simulink library "walkingRobotUtils"  (R2019b)
settings: Solver=VariableStepAuto  StartTime=0.0  StopTime=10.0  RelTol=1e-3
undefined symbols (not defined in the file): ankle_servo_kd, ankle_servo_ki, ankle_servo_kp, deriv_filter_coeff, foot_x, foot_y, foot_z, height_plane, hip_servo_kd, hip_servo_ki, hip_servo_kp, init_angs_L, init_angs_R, init_height, joint_damping, knee_servo_kd, knee_servo_ki, knee_servo_kp, leg_width, lower_leg_length, max_torque, motion_time_constant, motor_constant, motor_inertia, motor_voltage, plane_x, plane_y, plane_z, torso_height, torso_length, torso_offset_height, torso_offset_length, torso_offset_x, torso_offset_z, torso_width, torso_x, torso_y, torso_z, upper_leg_length, X, Y, Z
libraries: sm_lib x116, nesl_utility x49, $bdroot x33, simulink x33, simulink_extras x32, fl_lib x7, ee_lib x3, Multibody_Multiphysics_Lib x1
(part 1 of 6)
settings Model: Creator=scastro  LastModifiedBy=scastro
settings DataIOCC: ReturnWorkspaceOutputs=off
settings DebuggingCC: ArithmeticOperatorsInVariantConditions=warning
settings SFSimCC: SimUseLocalCustomCode=off  CustomCodeUndefinedFunction=UseInterfaceOnly
settings RTWCC: RTWUseLocalCustomCode=off
settings CodeAppCC: StateflowObjectComments=on

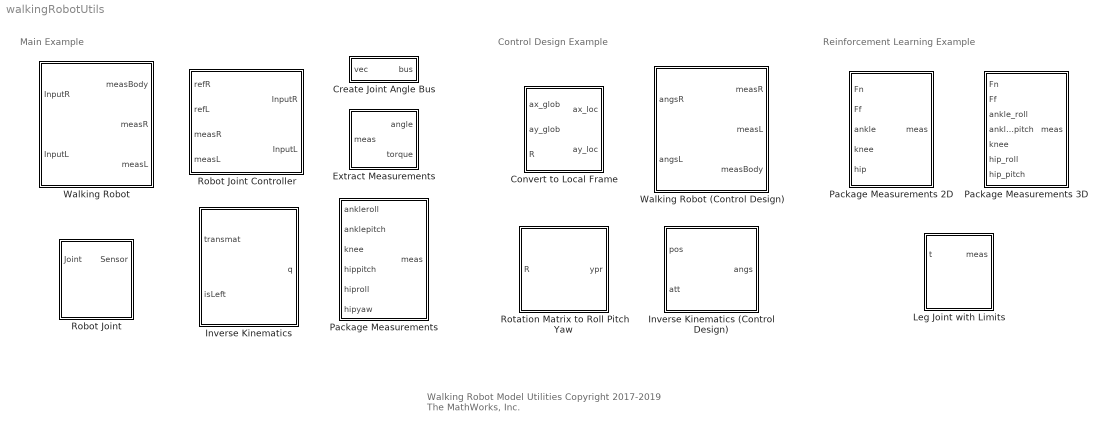
== system walkingRobotUtils ==
  note: Reinforcement Learning Example
  note: Control Design Example
  note: Main Example
  note: Walking Robot Model Utilities
      |
      | Copyright 2017-2019 The MathWorks, Inc.
  Convert to Local Frame : Subsystem
  Create Joint Angle Bus : Subsystem
  Extract Measurements : Subsystem
  Inverse Kinematics : MATLAB Function  TreatAsAtomicUnit=on
  Inverse Kinematics (Control Design) : MATLAB Function  TreatAsAtomicUnit=on
  Leg Joint with Limits : Subsystem  VariantControl=actuatorType == 2  mask(Leg Joint with Limits){k=1, d=0, initAngle=0, eqAngle=0, upperLimit=0, lowerLimit=-pi/8, jointLimitStiffness=100, jointLimitDamping=10}
      mask prompts: k "Joint Stiffness [N*m/rad]"; d "Joint Damping [N*m/(rad/s)]"; initAngle "Initial Angle [rad]"; eqAngle "Equilibrium Angle [rad]"; upperLimit "Upper Angle Limit [rad]"; lowerLimit "Lower Angle Limit [rad]"; jointLimitStiffness "Joint Limit Stiffness [N*m/rad]"; jointLimitDamping "Joint Limit Damping [N*m/(rad/s)]"
      mask help: Torque-actuated revolute joint with limits and instrumented measurements.
      mask DialogControl DynamicsTab Prompt: Dynamics
      mask DialogControl LimitsTab Prompt: Limits
  Package Measurements 3D : Subsystem
  Package Measurements 2D : Subsystem
  Package Measurements : Subsystem
  Robot Joint : Subsystem  Variant=on  mask{jointDamping=joint_damping, initAngle=0, upperLimit=pi/2, lowerLimit=-pi/2, limitK=1000, limitD=100}
      mask prompts: jointDamping "Joint Damping [N*m/(rad/s)"; initAngle "Initial Angle [rad]"; upperLimit "Upper Angle Limit [rad]"; lowerLimit "Lower Angle Limit [rad]"; limitK "Joint Limit Stiffness [N*m/rad]"; limitD "Joint Limit Damping [N*m/(rad/s)"
      mask help: Joint and actuator for walking robot example.
  Robot Joint Controller : Subsystem  Variant=on
  Rotation Matrix to Roll Pitch Yaw : MATLAB Function  TreatAsAtomicUnit=on
  Walking Robot : Subsystem
  Walking Robot (Control Design) : Subsystem

== system walkingRobotUtils/Convert to Local Frame ==
  ax_glob : Inport
  ay_glob : Inport  Port=2
  R : Inport  Port=3
  Constant : Constant  Value=0
  Demux1 : Demux  Outputs=2
  Matrix Multiply : Product  Multiplication=Matrix(*)
  Mux : Mux  Inputs=3
  Selector : Selector  InputPortWidth=3  IndexOptions=Index vector (dialog)  Indices=[1 2]  OutputSizes=1
  Transpose : Math  Operator=transpose  SaturateOnIntegerOverflow=on
  ax_loc : Outport  VectorParamsAs1DForOutWhenUnconnected=off
  ay_loc : Outport  Port=2  VectorParamsAs1DForOutWhenUnconnected=off
  wires:
  Mux/1 -> Matrix Multiply/2
  Demux1/2 -> ay_loc/1
  ay_glob/1 -> Mux/2
  Selector/1 -> Demux1/1
  Matrix Multiply/1 -> Selector/1
  Constant/1 -> Mux/3
  ax_glob/1 -> Mux/1
  Demux1/1 -> ax_loc/1
  R/1 -> Transpose/1
  Transpose/1 -> Matrix Multiply/1

== system walkingRobotUtils/Create Joint Angle Bus ==
  vec : Inport
  Bus Creator : BusCreator  Inputs=6
  Demux : Demux  Outputs=6
  Gain : Gain  Gain=-1
  Gain1 : Gain  Gain=-1
  Gain2 : Gain  Gain=-1
  bus : Outport  VectorParamsAs1DForOutWhenUnconnected=off
  wires:
  Gain2/1 -> Bus Creator/5  "ankle pitch"
  Gain1/1 -> Bus Creator/4  "knee"
  Demux/5 -> Gain2/1
  vec/1 -> Demux/1
  Demux/4 -> Gain1/1
  Bus Creator/1 -> bus/1
  Gain/1 -> Bus Creator/3  "hip pitch"
  Demux/1 -> Bus Creator/1  "hip yaw"
  Demux/6 -> Bus Creator/6  "ankle roll"
  Demux/2 -> Bus Creator/2  "hip roll"
  Demux/3 -> Gain/1

== system walkingRobotUtils/Extract Measurements ==
  meas : Inport
  Bus Selector : BusSelector  OutputSignals=angle,torque
  angle : Outport  VectorParamsAs1DForOutWhenUnconnected=off
  torque : Outport  Port=2  VectorParamsAs1DForOutWhenUnconnected=off
  wires:
  Bus Selector/1 -> angle/1  "<angle>"
  meas/1 -> Bus Selector/1
  Bus Selector/2 -> torque/1  "<torque>"

== system walkingRobotUtils/Leg Joint with Limits ==
  t : Inport
  Bus Creator : BusCreator  Inputs=3
  PS-Simulink Converter1 : nesl_utility/PS-Simulink Converter  PhysicalDomain=network_engine_domain  SubClassName=ps_output  LeftPortType=input  RightPortType=output  PseudoPeriodic=off  Frequencies=[]  Unit=rad  AffineConversion=off
  PS-Simulink Converter2 : nesl_utility/PS-Simulink Converter  PhysicalDomain=network_engine_domain  SubClassName=ps_output  LeftPortType=input  RightPortType=output  PseudoPeriodic=off  Frequencies=[]  Unit=rad/s  AffineConversion=off
  Revolute Joint : sm_lib/Joints/Revolute Joint  JointMode=Normal  SenseConstraintForce=off  SenseConstraintForceX=off  SenseConstraintForceY=off  SenseConstraintForceZ=off  SenseConstraintTorque=off  SenseConstraintTorqueX=off  SenseConstraintTorqueY=off  SenseConstraintTorqueZ=off  SenseTotalForce=off  SenseTotalForceX=off  SenseTotalForceY=off  SenseTotalForceZ=off  SenseTotalTorque=off  SenseTotalTorqueX=off  SenseTotalTorqueY=off  SenseTotalTorqueZ=off  CompositeWrenchDir=FollowerOnBase  CompositeWrenchFrame=BaseFrame  EquilibriumPosition=eqAngle  EquilibriumPositionUnits=rad  SpringStiffness=k  SpringStiffnessUnits=N*m/rad  DampingCoefficient=d  DampingCoefficientUnits=N*m/(rad/s)  TorqueActuationMode=InputTorque  MotionActuationMode=ComputedMotion  SensePosition=on  SenseVelocity=on  SenseAcceleration=off  SenseTorqueForce=off  SenseLowerLimitTorqueForce=off  SenseUpperLimitTorqueForce=off  LowerLimitSpecify=on  LowerLimitBound=lowerLimit  LowerLimitBoundUnits=rad  LowerLimitStiffness=jointLimitStiffness  LowerLimitStiffnessUnits=N*m/rad  LowerLimitDamping=jointLimitDamping  LowerLimitDampingUnits=N*m/(rad/s)  LowerLimitTransitionRegionWidth=1  LowerLimitTransitionRegionWidthUnits=deg  UpperLimitSpecify=on  UpperLimitBound=upperLimit  UpperLimitBoundUnits=rad  UpperLimitStiffness=jointLimitStiffness  UpperLimitStiffnessUnits=N*m/rad  UpperLimitDamping=jointLimitDamping  UpperLimitDampingUnits=N*m/(rad/s)  UpperLimitTransitionRegionWidth=1  UpperLimitTransitionRegionWidthUnits=deg  PositionTargetSpecify=on  PositionTargetPriority=High  PositionTargetValue=initAngle  PositionTargetValueUnits=rad  VelocityTargetSpecify=off  VelocityTargetPriority=High  VelocityTargetValue=0  VelocityTargetValueUnits=deg/s
  Simulink-PS Converter : nesl_utility/Simulink-PS Converter  PhysicalDomain=network_engine_domain  SubClassName=ps_input  LeftPortType=input  RightPortType=output  PseudoPeriodic=off  Frequencies=[]  NoiseDistribution=none  NoiseParameters=[]  Unit=N*m  AffineConversion=off  FilteringAndDerivatives=provide  SimscapeFilterOrder=2  InputFilterTimeConstant=motion_time_constant  UdotUserProvided=0
  B : PMIOPort  Side=Left
  F : PMIOPort  Port=2  Side=Right
  meas : Outport  VectorParamsAs1DForOutWhenUnconnected=off
  wires:
  PS-Simulink Converter2/1 -> Bus Creator/3  "speed"
  t/1 -> Simulink-PS Converter/1, Bus Creator/1  "torque"
  Bus Creator/1 -> meas/1
  PS-Simulink Converter1/1 -> Bus Creator/2  "angle"
  connections:
  PS-Simulink Converter2/LConn1 -- Revolute Joint/RConn3
  Simulink-PS Converter/RConn1 -- Revolute Joint/LConn2
  Revolute Joint/RConn1 -- F/RConn1
  Revolute Joint/LConn1 -- B/RConn1
  PS-Simulink Converter1/LConn1 -- Revolute Joint/RConn2

== system walkingRobotUtils/Package Measurements 3D ==
  Fn : Inport
  Ff : Inport  Port=2
  ankle_roll : Inport  Port=3
  ankle_pitch : Inport  Port=4
  knee : Inport  Port=5
  hip_roll : Inport  Port=6
  hip_pitch : Inport  Port=7
  Bus Creator3 : BusCreator  Inputs=17
  Extract Measurements : Subsystem
  Extract Measurements1 : Subsystem
  Extract Measurements2 : Subsystem
  Extract Measurements3 : Subsystem
  Extract Measurements4 : Subsystem
  meas : Outport  VectorParamsAs1DForOutWhenUnconnected=off
  wires:
  Extract Measurements4/2(speed) -> Bus Creator3/16  "hip_pitch_speed"
  Extract Measurements3/2(speed) -> Bus Creator3/13  "hip_roll_speed"
  Extract Measurements2/2(speed) -> Bus Creator3/10  "knee_speed"
  Extract Measurements2/1(angle) -> Bus Creator3/9  "knee_angle"
  Extract Measurements1/2(speed) -> Bus Creator3/7  "ankle_pitch_speed"
  Extract Measurements/2(speed) -> Bus Creator3/4  "ankle_roll_speed"
  Fn/1 -> Bus Creator3/1  "normal_force"
  Ff/1 -> Bus Creator3/2  "friction_force"
  Extract Measurements4/3(torque) -> Bus Creator3/17  "hip_pitch_torque"
  Extract Measurements4/1(angle) -> Bus Creator3/15  "hip_pitch_angle"
  Extract Measurements2/3(torque) -> Bus Creator3/11  "knee_torque"
  hip_pitch/1 -> Extract Measurements4/1(meas)
  knee/1 -> Extract Measurements2/1(meas)
  Extract Measurements1/3(torque) -> Bus Creator3/8  "ankle_pitch_torque"
  Extract Measurements1/1(angle) -> Bus Creator3/6  "ankle_pitch_angle"
  ankle_pitch/1 -> Extract Measurements1/1(meas)
  Bus Creator3/1 -> meas/1
  ankle_roll/1 -> Extract Measurements/1(meas)
  Extract Measurements/1(angle) -> Bus Creator3/3  "ankle_roll_angle"
  Extract Measurements/3(torque) -> Bus Creator3/5  "ankle_roll_torque"
  hip_roll/1 -> Extract Measurements3/1(meas)
  Extract Measurements3/3(torque) -> Bus Creator3/14  "hip_roll_torque"
  Extract Measurements3/1(angle) -> Bus Creator3/12  "hip_roll_angle"

== system walkingRobotUtils/Package Measurements 2D ==
  Fn : Inport
  Ff : Inport  Port=2
  ankle : Inport  Port=3
  knee : Inport  Port=4
  hip : Inport  Port=5
  Bus Creator3 : BusCreator  Inputs=11
  Extract Measurements : Subsystem
  Extract Measurements1 : Subsystem
  Extract Measurements2 : Subsystem
  meas : Outport  VectorParamsAs1DForOutWhenUnconnected=off
  wires:
  Extract Measurements2/2(speed) -> Bus Creator3/10  "hip_speed"
  Extract Measurements1/2(speed) -> Bus Creator3/7  "knee_speed"
  Extract Measurements/2(speed) -> Bus Creator3/4  "ankle_speed"
  Bus Creator3/1 -> meas/1
  ankle/1 -> Extract Measurements/1(meas)
  Extract Measurements/1(angle) -> Bus Creator3/3  "ankle_angle"
  Extract Measurements/3(torque) -> Bus Creator3/5  "ankle_torque"
  knee/1 -> Extract Measurements1/1(meas)
  hip/1 -> Extract Measurements2/1(meas)
  Extract Measurements1/1(angle) -> Bus Creator3/6  "knee_angle"
  Extract Measurements1/3(torque) -> Bus Creator3/8  "knee_torque"
  Extract Measurements2/1(angle) -> Bus Creator3/9  "hip_angle"
  Extract Measurements2/3(torque) -> Bus Creator3/11  "hip_torque"
  Ff/1 -> Bus Creator3/2  "friction_force"
  Fn/1 -> Bus Creator3/1  "normal_force"

== system walkingRobotUtils/Package Measurements ==
  ankleroll : Inport
  anklepitch : Inport  Port=2
  knee : Inport  Port=3
  hippitch : Inport  Port=4
  hiproll : Inport  Port=5
  hipyaw : Inport  Port=6
  Bus Creator3 : BusCreator  Inputs=12
  Extract Measurements : Subsystem
  Extract Measurements{1..5} (5 alike) : $bdroot/Package Measurements/Extract Measurements  SystemSampleTime=-1  Latency=0  AutoFrameSizeCalculation=off
  meas : Outport  VectorParamsAs1DForOutWhenUnconnected=off
  wires:
  hiproll/1 -> Extract Measurements4/1
  Extract Measurements1/2 -> Bus Creator3/4  "anklepitch_torque"
  Bus Creator3/1 -> meas/1
  anklepitch/1 -> Extract Measurements1/1
  hippitch/1 -> Extract Measurements3/1
  hipyaw/1 -> Extract Measurements5/1
  Extract Measurements5/1 -> Bus Creator3/11  "hipyaw_angle"
  Extract Measurements/2(torque) -> Bus Creator3/2  "ankleroll_torque"
  Extract Measurements4/1 -> Bus Creator3/9  "hiproll_angle"
  knee/1 -> Extract Measurements2/1
  Extract Measurements2/1 -> Bus Creator3/5  "knee_angle"
  Extract Measurements/1(angle) -> Bus Creator3/1  "ankleroll_angle"
  ankleroll/1 -> Extract Measurements/1(meas)
  Extract Measurements3/2 -> Bus Creator3/8  "hippitch_torque"
  Extract Measurements1/1 -> Bus Creator3/3  "anklepitch_angle"
  Extract Measurements3/1 -> Bus Creator3/7  "hippitch_angle"
  Extract Measurements5/2 -> Bus Creator3/12  "hipyaw_torque"
  Extract Measurements2/2 -> Bus Creator3/6  "knee_torque"
  Extract Measurements4/2 -> Bus Creator3/10  "hiproll_torque"

== system walkingRobotUtils/Robot Joint ==
  note: 1) Add Subsystem or Model blocks as valid variant choices.
      | 2) You cannot connect blocks at this level. At simulation, connectivity is automatically
      | determined, based on the active variant and port name matching.
  Joint : Inport
  Motion : Subsystem  VariantControl=actuatorType == 1
  Motor : Subsystem  VariantControl=actuatorType == 3
  Torque : Subsystem  VariantControl=actuatorType == 2
  F : PMIOPort  Side=Right
  B : PMIOPort  Port=2  Side=Left
  Sensor : Outport  VectorParamsAs1DForOutWhenUnconnected=off

== system walkingRobotUtils/Robot Joint Controller ==
  note: 1) Add Subsystem or Model blocks as valid variant choices.
      | 2) You cannot connect blocks at this level. At simulation, connectivity is automatically
      | determined, based on the active variant and port name matching.
  refR : Inport
  refL : Inport  Port=2
  measR : Inport  Port=3
  measL : Inport  Port=4
  Motion : Subsystem  VariantControl=actuatorType == 1
  Motor : Subsystem  VariantControl=actuatorType == 3
  Torque : Subsystem  VariantControl=actuatorType == 2
  InputR : Outport  VectorParamsAs1DForOutWhenUnconnected=off
  InputL : Outport  Port=2  VectorParamsAs1DForOutWhenUnconnected=off

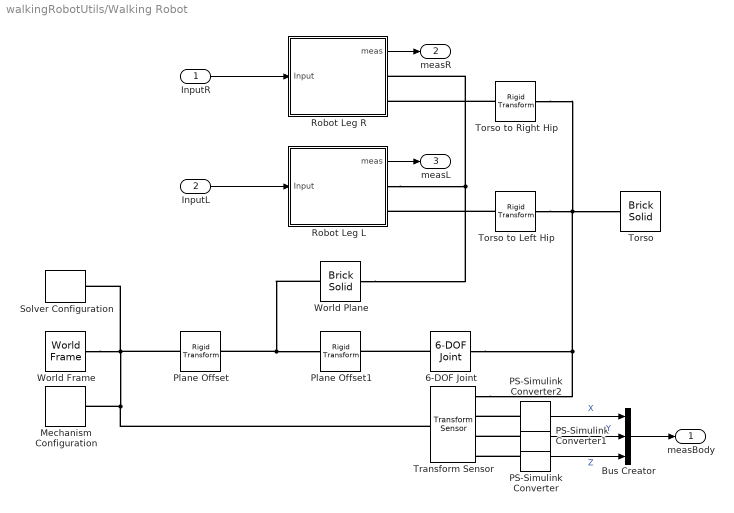
== system walkingRobotUtils/Walking Robot ==
  InputR : Inport
  InputL : Inport  Port=2
  6-DOF Joint : sm_lib/Joints/6-DOF Joint  JointMode=Normal  SenseConstraintForce=off  SenseConstraintForceX=off  SenseConstraintForceY=off  SenseConstraintForceZ=off  SenseConstraintTorque=off  SenseConstraintTorqueX=off  SenseConstraintTorqueY=off  SenseConstraintTorqueZ=off  SenseTotalForce=off  SenseTotalForceX=off  SenseTotalForceY=off  SenseTotalForceZ=off  SenseTotalTorque=off  SenseTotalTorqueX=off  SenseTotalTorqueY=off  SenseTotalTorqueZ=off  CompositeWrenchDir=FollowerOnBase  CompositeWrenchFrame=BaseFrame  PxEquilibriumPosition=0  PxEquilibriumPositionUnits=m  PxSpringStiffness=0  PxSpringStiffnessUnits=N/m  PxDampingCoefficient=world_damping  PxDampingCoefficientUnits=N/(m/s)  PxTorqueActuationMode=NoTorque  PxMotionActuationMode=ComputedMotion  PxSensePosition=off  PxSenseVelocity=off  PxSenseAcceleration=off  PxSenseTorqueForce=off  PxSenseLowerLimitTorqueForce=off  PxSenseUpperLimitTorqueForce=off  PxLowerLimitSpecify=off  PxLowerLimitBound=-1  PxLowerLimitBoundUnits=m  PxLowerLimitStiffness=1e6  PxLowerLimitStiffnessUnits=N/m  PxLowerLimitDamping=1e3  PxLowerLimitDampingUnits=N/(m/s)  PxLowerLimitTransitionRegionWidth=1e-4  PxLowerLimitTransitionRegionWidthUnits=m  PxUpperLimitSpecify=off  PxUpperLimitBound=1  PxUpperLimitBoundUnits=m  PxUpperLimitStiffness=1e6  PxUpperLimitStiffnessUnits=N/m  PxUpperLimitDamping=1e3  PxUpperLimitDampingUnits=N/(m/s)  PxUpperLimitTransitionRegionWidth=1e-4  PxUpperLimitTransitionRegionWidthUnits=m  PxPositionTargetSpecify=off  PxPositionTargetPriority=High  PxPositionTargetValue=0  PxPositionTargetValueUnits=m  PxVelocityTargetSpecify=off  PxVelocityTargetPriority=High  PxVelocityTargetValue=0  PxVelocityTargetValueUnits=m/s  PyEquilibriumPosition=0  PyEquilibriumPositionUnits=m  PySpringStiffness=0  PySpringStiffnessUnits=N/m  PyDampingCoefficient=world_damping  PyDampingCoefficientUnits=N/(m/s)  PyTorqueActuationMode=NoTorque  PyMotionActuationMode=ComputedMotion  PySensePosition=off  PySenseVelocity=off  PySenseAcceleration=off  PySenseTorqueForce=off  PySenseLowerLimitTorqueForce=off  PySenseUpperLimitTorqueForce=off  PyLowerLimitSpecify=off  PyLowerLimitBound=-1  PyLowerLimitBoundUnits=m  PyLowerLimitStiffness=1e6  PyLowerLimitStiffnessUnits=N/m  PyLowerLimitDamping=1e3  PyLowerLimitDampingUnits=N/(m/s)  PyLowerLimitTransitionRegionWidth=1e-4  PyLowerLimitTransitionRegionWidthUnits=m  PyUpperLimitSpecify=off  PyUpperLimitBound=1  PyUpperLimitBoundUnits=m  PyUpperLimitStiffness=1e6  PyUpperLimitStiffnessUnits=N/m  PyUpperLimitDamping=1e3  PyUpperLimitDampingUnits=N/(m/s)  PyUpperLimitTransitionRegionWidth=1e-4  PyUpperLimitTransitionRegionWidthUnits=m  PyPositionTargetSpecify=off  PyPositionTargetPriority=High  PyPositionTargetValue=0  PyPositionTargetValueUnits=m  PyVelocityTargetSpecify=off  PyVelocityTargetPriority=High  PyVelocityTargetValue=0  PyVelocityTargetValueUnits=m/s  PzEquilibriumPosition=0  PzEquilibriumPositionUnits=m  PzSpringStiffness=0  PzSpringStiffnessUnits=N/m  PzDampingCoefficient=world_damping  PzDampingCoefficientUnits=N/(m/s)  PzTorqueActuationMode=NoTorque  PzMotionActuationMode=ComputedMotion  PzSensePosition=off  PzSenseVelocity=off  PzSenseAcceleration=off  PzSenseTorqueForce=off  PzSenseLowerLimitTorqueForce=off  PzSenseUpperLimitTorqueForce=off  PzLowerLimitSpecify=off  PzLowerLimitBound=-1  PzLowerLimitBoundUnits=m  PzLowerLimitStiffness=1e6  PzLowerLimitStiffnessUnits=N/m  PzLowerLimitDamping=1e3  PzLowerLimitDampingUnits=N/(m/s)  PzLowerLimitTransitionRegionWidth=1e-4  PzLowerLimitTransitionRegionWidthUnits=m  PzUpperLimitSpecify=off  PzUpperLimitBound=1  PzUpperLimitBoundUnits=m  PzUpperLimitStiffness=1e6  PzUpperLimitStiffnessUnits=N/m  PzUpperLimitDamping=1e3  PzUpperLimitDampingUnits=N/(m/s)  PzUpperLimitTransitionRegionWidth=1e-4  PzUpperLimitTransitionRegionWidthUnits=m  PzPositionTargetSpecify=on  PzPositionTargetPriority=High  PzPositionTargetValue=init_height  PzPositionTargetValueUnits=m  PzVelocityTargetSpecify=off  PzVelocityTargetPriority=High  PzVelocityTargetValue=0  PzVelocityTargetValueUnits=m/s  SphDefPosRotationMethod=None  SphDefPosRotationAngleUnits=deg  SphDefPosRotationStandardAxis=+Z  SphDefPosRotationAngle=0.0  SphDefPosRotationArbitraryAxis=[0 0 1]  SphDefPosFollAlignAxisA=+X  SphDefPosBaseAlignAxisA=+Y  SphDefPosFollAlignAxisB=+Y  SphDefPosBaseAlignAxisB=+Z  SphDefPosRotationSequenceAxes=FollowerAxes  SphDefPosRotationSequence=XYX  SphDefPosRotationSequenceAngles=[0 0 0]  SphDefPosRotationSequenceAnglesUnits=deg  SphDefPosRotationMatrix=[1 0 0; 0 1 0; 0 0 1]  SphEqPosRotationMethod=None  SphEqPosRotationAngleUnits=deg  SphEqPosRotationStandardAxis=+Z  SphEqPosRotationAngle=0.0  SphEqPosRotationArbitraryAxis=[0 0 1]  SphEqPosFollAlignAxisA=+X  SphEqPosBaseAlignAxisA=+Y  SphEqPosFollAlignAxisB=+Y  SphEqPosBaseAlignAxisB=+Z  SphEqPosRotationSequenceAxes=FollowerAxes  SphEqPosRotationSequence=XYX  SphEqPosRotationSequenceAngles=[0 0 0]  SphEqPosRotationSequenceAnglesUnits=deg  SphEqPosRotationMatrix=[1 0 0; 0 1 0; 0 0 1]  SphSpringStiffness=0  SphSpringStiffnessUnits=N*m/deg  SphDampingCoefficient=world_rot_damping  SphDampingCoefficientUnits=N*m/(rad/s)  SphActuateTorqueX=off  SphActuateTorqueY=off  SphActuateTorqueZ=off  SphActuateTorque=off  SphTorqueActuationMode=NoTorque  SphMotionActuationMode=ComputedMotion  SphActuationFrame=BaseFrame  SphSensePosition=off  SphSenseVelocityX=off  SphSenseVelocityY=off  SphSenseVelocityZ=off  SphSenseVelocity=off  SphSenseAccelerationX=off  SphSenseAccelerationY=off  SphSenseAccelerationZ=off  SphSenseAcceleration=off  SphSenseTorqueX=off  SphSenseTorqueY=off  SphSenseTorqueZ=off  SphSenseTorqueForce=off  SphSenseLowerLimitTorqueMag=off  SphSenseUpperLimitTorqueMag=off  SphSensingFrame=BaseFrame  SphLowerLimitSpecify=off  SphLowerLimitBound=15  SphLowerLimitBoundUnits=deg  SphLowerLimitStiffness=1e4  SphLowerLimitStiffnessUnits=N*m/deg  SphLowerLimitDamping=10  SphLowerLimitDampingUnits=N*m/(deg/s)  SphLowerLimitTransitionRegionWidth=0.1  SphLowerLimitTransitionRegionWidthUnits=deg  SphUpperLimitSpecify=off  SphUpperLimitBound=45  SphUpperLimitBoundUnits=deg  SphUpperLimitStiffness=1e4  SphUpperLimitStiffnessUnits=N*m/deg  SphUpperLimitDamping=10  SphUpperLimitDampingUnits=N*m/(deg/s)  SphUpperLimitTransitionRegionWidth=0.1  SphUpperLimitTransitionRegionWidthUnits=deg  SphPositionTargetRotationMethod=None  SphPositionTargetRotationAngleUnits=deg  SphPositionTargetRotationStandardAxis=+Z  SphPositionTargetRotationAngle=0.0  SphPositionTargetRotationArbitraryAxis=[0 0 1]  SphPositionTargetFollAlignAxisA=+X  SphPositionTargetBaseAlignAxisA=+Y  SphPositionTargetFollAlignAxisB=+Y  SphPositionTargetBaseAlignAxisB=+Z  SphPositionTargetRotationSequenceAxes=FollowerAxes  SphPositionTargetRotationSequence=XYX  SphPositionTargetRotationSequenceAngles=[0 0 0]  SphPositionTargetRotationSequenceAnglesUnits=deg  SphPositionTargetRotationMatrix=[1 0 0; 0 1 0; 0 0 1]  SphPositionTargetSpecify=off  SphPositionTargetPriority=High  SphVelocityTargetValue=[0 0 0]  SphVelocityTargetValueUnits=deg/s  SphVelocityTargetSpecify=off  SphVelocityTargetPriority=High  SphVelocityTargetInFollowerFrame=on
  Bus Creator : BusCreator  Inputs=3
  Mechanism Configuration : sm_lib/Utilities/Mechanism Configuration  UniformGravity=Constant  GravityVector=[0 0 -9.80665]  GravityUnits=m/s^2  LinearizationDelta=0.001
  PS-Simulink Converter : nesl_utility/PS-Simulink Converter  PhysicalDomain=network_engine_domain  SubClassName=ps_output  LeftPortType=input  RightPortType=output  PseudoPeriodic=off  Frequencies=[]  Unit=m  AffineConversion=off
  PS-Simulink Converter1 : nesl_utility/PS-Simulink Converter  PhysicalDomain=network_engine_domain  SubClassName=ps_output  LeftPortType=input  RightPortType=output  PseudoPeriodic=off  Frequencies=[]  Unit=m  AffineConversion=off
  PS-Simulink Converter2 : nesl_utility/PS-Simulink Converter  PhysicalDomain=network_engine_domain  SubClassName=ps_output  LeftPortType=input  RightPortType=output  PseudoPeriodic=off  Frequencies=[]  Unit=m  AffineConversion=off
  Plane Offset : sm_lib/Frames and Transforms/Rigid Transform  TranslationMethod=StandardAxis  TranslationStandardOffset=plane_z/2  TranslationLengthUnit=m  TranslationStandardAxis=-Z  TranslationCartesianOffset=[0 0 0]  TranslationROffset=0  TranslationROffsetUnits=m  TranslationZOffset=0  TranslationZOffsetUnits=m  TranslationThetaOffset=0  TranslationThetaOffsetUnits=deg  RotationMethod=None  RotationAngleUnits=deg  RotationStandardAxis=+Z  RotationAngle=0.0  RotationArbitraryAxis=[0 0 1]  FollAlignAxisA=+X  BaseAlignAxisA=+Y  FollAlignAxisB=+Y  BaseAlignAxisB=+Z  RotationSequenceAxes=FollowerAxes  RotationSequence=XYX  RotationSequenceAngles=[0 0 0]  RotationSequenceAnglesUnits=deg  RotationMatrix=[1 0 0; 0 1 0; 0 0 1]
  Plane Offset1 : sm_lib/Frames and Transforms/Rigid Transform  TranslationMethod=StandardAxis  TranslationStandardOffset=plane_z/2  TranslationLengthUnit=m  TranslationStandardAxis=+Z  TranslationCartesianOffset=[0 0 0]  TranslationROffset=0  TranslationROffsetUnits=m  TranslationZOffset=0  TranslationZOffsetUnits=m  TranslationThetaOffset=0  TranslationThetaOffsetUnits=deg  RotationMethod=None  RotationAngleUnits=deg  RotationStandardAxis=+Z  RotationAngle=0.0  RotationArbitraryAxis=[0 0 1]  FollAlignAxisA=+X  BaseAlignAxisA=+Y  FollAlignAxisB=+Y  BaseAlignAxisB=+Z  RotationSequenceAxes=FollowerAxes  RotationSequence=XYX  RotationSequenceAngles=[0 0 0]  RotationSequenceAnglesUnits=deg  RotationMatrix=[1 0 0; 0 1 0; 0 0 1]
  Robot Leg L : Subsystem
  Robot Leg R : Subsystem
  Solver Configuration : nesl_utility/Solver Configuration  PhysicalDomain=network_engine_domain  SubClassName=solver  LeftPortType=input  RightPortType=generic  Tones=[]  Harmonics=[]  SimulateNoise=off  Profile=off  UseLocalSampling=off  EnableSwitchedLinearOptims=on  FrequencyDomain=off  UseCCode=off  RelTol=0.001  AbsTol=1e-06  MinStep=1e-09  ToWorkspace=off  RevertToSquareIcSolve=off  NumHomotopyIterations=100  PhasorMode=off  PhasorModeNumHarmonics=1  DoDC=off  ResidualTolerance=1e-09  UseLocalSolver=off  LocalSolverChoice=NE_TRAPEZOIDAL_ADVANCER  LocalSolverSampleTime=0.001  DoFixedCost=off  MaxNonlinIter=3  MaxModeIter=2  LinearAlgebra=Sparse  EquationFormulation=NE_TIME_EF  DelaysMemoryBudget=1024  AutomaticFiltering=on  FilteringTimeConstant=0.001  PartitionStorageMethod=AS_NEEDED  PartitionMemoryBudget=1024  PartitionMethod=FAST
  Torso : sm_lib/Body Elements/Brick Solid  GraphicAmbientColor=[0.15 0.15 0.15 1.0]  BasedOnType=Density  BrickDimensions=[torso_width torso_length torso_height]  BrickDimensionUnits=m  CenterOfMass=[0 0 0]  CenterOfMassUnits=m  GraphicDiffuseColor=[0.5 0.5 0.5]  Density=1000  DensityUnits=kg/m^3  DoExposeReferenceFrame=on  GraphicEmissiveColor=[0.0 0.0 0.0 1.0]  ExportEntireGeometry=off  SerializedFrames=<Frames/>  MarkerShape=Sphere  MarkerSize=10  GraphicType=FromGeometry  InertiaType=CalculateFromGeometry  Mass=1  MassUnits=kg  MomentsOfInertia=[1 1 1]  MomentsOfInertiaUnits=kg*m^2  GraphicOpacity=1.0  ProductsOfInertia=[1 1 1]  ProductsOfInertiaUnits=kg*m^2  GraphicShininess=75  GraphicSpecularColor=[0.5 0.5 0.5 1.0]  GraphicVisPropType=SimpleVisualProperties
  Torso to Left Hip : sm_lib/Frames and Transforms/Rigid Transform  TranslationMethod=Cartesian  TranslationStandardOffset=0  TranslationLengthUnit=m  TranslationStandardAxis=+Z  TranslationCartesianOffset=[-torso_width/2 torso_offset_length torso_offset_height]  TranslationROffset=0  TranslationROffsetUnits=m  TranslationZOffset=0  TranslationZOffsetUnits=m  TranslationThetaOffset=0  TranslationThetaOffsetUnits=deg  RotationMethod=None  RotationAngleUnits=deg  RotationStandardAxis=+Z  RotationAngle=0.0  RotationArbitraryAxis=[0 0 1]  FollAlignAxisA=+X  BaseAlignAxisA=+Y  FollAlignAxisB=+Y  BaseAlignAxisB=+Z  RotationSequenceAxes=FollowerAxes  RotationSequence=XYX  RotationSequenceAngles=[0 0 0]  RotationSequenceAnglesUnits=deg  RotationMatrix=[1 0 0; 0 1 0; 0 0 1]
  Torso to Right Hip : sm_lib/Frames and Transforms/Rigid Transform  TranslationMethod=Cartesian  TranslationStandardOffset=0  TranslationLengthUnit=m  TranslationStandardAxis=+Z  TranslationCartesianOffset=[torso_width/2 torso_offset_length torso_offset_height]  TranslationROffset=0  TranslationROffsetUnits=m  TranslationZOffset=0  TranslationZOffsetUnits=m  TranslationThetaOffset=0  TranslationThetaOffsetUnits=deg  RotationMethod=None  RotationAngleUnits=deg  RotationStandardAxis=+Z  RotationAngle=0.0  RotationArbitraryAxis=[0 0 1]  FollAlignAxisA=+X  BaseAlignAxisA=+Y  FollAlignAxisB=+Y  BaseAlignAxisB=+Z  RotationSequenceAxes=FollowerAxes  RotationSequence=XYX  RotationSequenceAngles=[0 0 0]  RotationSequenceAnglesUnits=deg  RotationMatrix=[1 0 0; 0 1 0; 0 0 1]
  Transform Sensor : sm_lib/Frames and Transforms/Transform Sensor  MeasurementFrame=World  SenseAngle=off  SenseAxis=off  SenseAngle1=off  SenseAngle2=off  SenseAngle3=off  SenseQ=off  SenseR=off  SenseOmegaX=off  SenseOmegaY=off  SenseOmegaZ=off  SenseOmega1=off  SenseOmega2=off  SenseOmega3=off  SenseQDot=off  SenseRDot=off  SenseAlphaX=off  SenseAlphaY=off  SenseAlphaZ=off  SenseAlpha1=off  SenseAlpha2=off  SenseAlpha3=off  SenseQDDot=off  SenseRDDot=off  SenseX=on  SenseY=on  SenseZ=on  SenseRad=off  SenseAzim=off  SenseDist=off  SenseInc=off  SenseXDot=off  SenseYDot=off  SenseZDot=off  SenseRadDot=off  SenseAzimDot=off  SenseDistDot=off  SenseIncDot=off  SenseXDDot=off  SenseYDDot=off  SenseZDDot=off  SenseRadDDot=off  SenseAzimDDot=off  SenseDistDDot=off  SenseIncDDot=off
  World Frame : sm_lib/Frames and Transforms/World Frame
  World Plane : sm_lib/Body Elements/Brick Solid  GraphicAmbientColor=[0.15 0.15 0.15 1.0]  BasedOnType=Density  BrickDimensions=[plane_x plane_y plane_z]  BrickDimensionUnits=m  CenterOfMass=[0 0 0]  CenterOfMassUnits=m  GraphicDiffuseColor=[1.0 1.0 0.8]  Density=1000  DensityUnits=kg/(m^3)  DoExposeReferenceFrame=on  GraphicEmissiveColor=[0.0 0.0 0.0 1.0]  ExportEntireGeometry=on  SerializedFrames=<Frames/>  MarkerShape=Sphere  MarkerSize=10  GraphicType=FromGeometry  InertiaType=CalculateFromGeometry  Mass=1  MassUnits=kg  MomentsOfInertia=[1 1 1]  MomentsOfInertiaUnits=kg*m^2  GraphicOpacity=0.5  ProductsOfInertia=[0 0 0]  ProductsOfInertiaUnits=kg*m^2  GraphicShininess=75  GraphicSpecularColor=[0.5 0.5 0.5 1.0]  GraphicVisPropType=SimpleVisualProperties
  measBody : Outport  VectorParamsAs1DForOutWhenUnconnected=off
  measR : Outport  Port=2  VectorParamsAs1DForOutWhenUnconnected=off
  measL : Outport  Port=3  VectorParamsAs1DForOutWhenUnconnected=off
  wires:
  Robot Leg L/1(meas) -> measL/1
  Robot Leg R/1(meas) -> measR/1
  InputR/1 -> Robot Leg R/1(Input)
  InputL/1 -> Robot Leg L/1(Input)
  PS-Simulink Converter1/1 -> Bus Creator/2  "Y"
  PS-Simulink Converter2/1 -> Bus Creator/1  "X"
  PS-Simulink Converter/1 -> Bus Creator/3  "Z"
  Bus Creator/1 -> measBody/1
  connections:
  Torso to Right Hip/RConn1 -- Robot Leg R/RConn2
  Torso to Left Hip/RConn1 -- Robot Leg L/RConn2
  Robot Leg L/RConn1 -- World Plane/LConn1 -- Robot Leg R/RConn1
  Torso to Right Hip/LConn1 -- 6-DOF Joint/RConn1 -- Transform Sensor/RConn1 -- Torso/RConn1 -- Torso to Left Hip/LConn1
  Solver Configuration/RConn1 -- Plane Offset/LConn1 -- World Frame/RConn1 -- Transform Sensor/LConn1 -- Mechanism Configuration/RConn1
  6-DOF Joint/LConn1 -- Plane Offset1/RConn1
  World Plane/RConn1 -- Plane Offset1/LConn1 -- Plane Offset/RConn1
  PS-Simulink Converter1/LConn1 -- Transform Sensor/RConn3
  PS-Simulink Converter2/LConn1 -- Transform Sensor/RConn2
  PS-Simulink Converter/LConn1 -- Transform Sensor/RConn4

== system walkingRobotUtils/Walking Robot (Control Design) ==
  angsR : Inport
  angsL : Inport  Port=2
  6-DOF Joint : sm_lib/Joints/6-DOF Joint  JointMode=Normal  SenseConstraintForce=off  SenseConstraintForceX=off  SenseConstraintForceY=off  SenseConstraintForceZ=off  SenseConstraintTorque=off  SenseConstraintTorqueX=off  SenseConstraintTorqueY=off  SenseConstraintTorqueZ=off  SenseTotalForce=off  SenseTotalForceX=off  SenseTotalForceY=off  SenseTotalForceZ=off  SenseTotalTorque=off  SenseTotalTorqueX=off  SenseTotalTorqueY=off  SenseTotalTorqueZ=off  CompositeWrenchDir=FollowerOnBase  CompositeWrenchFrame=BaseFrame  PxEquilibriumPosition=0  PxEquilibriumPositionUnits=m  PxSpringStiffness=0  PxSpringStiffnessUnits=N/m  PxDampingCoefficient=world_damping  PxDampingCoefficientUnits=N/(m/s)  PxTorqueActuationMode=NoTorque  PxMotionActuationMode=ComputedMotion  PxSensePosition=off  PxSenseVelocity=off  PxSenseAcceleration=off  PxSenseTorqueForce=off  PxSenseLowerLimitTorqueForce=off  PxSenseUpperLimitTorqueForce=off  PxLowerLimitSpecify=off  PxLowerLimitBound=-1  PxLowerLimitBoundUnits=m  PxLowerLimitStiffness=1e6  PxLowerLimitStiffnessUnits=N/m  PxLowerLimitDamping=1e3  PxLowerLimitDampingUnits=N/(m/s)  PxLowerLimitTransitionRegionWidth=1e-4  PxLowerLimitTransitionRegionWidthUnits=m  PxUpperLimitSpecify=off  PxUpperLimitBound=1  PxUpperLimitBoundUnits=m  PxUpperLimitStiffness=1e6  PxUpperLimitStiffnessUnits=N/m  PxUpperLimitDamping=1e3  PxUpperLimitDampingUnits=N/(m/s)  PxUpperLimitTransitionRegionWidth=1e-4  PxUpperLimitTransitionRegionWidthUnits=m  PxPositionTargetSpecify=on  PxPositionTargetPriority=High  PxPositionTargetValue=0  PxPositionTargetValueUnits=m  PxVelocityTargetSpecify=off  PxVelocityTargetPriority=High  PxVelocityTargetValue=0  PxVelocityTargetValueUnits=m/s  PyEquilibriumPosition=0  PyEquilibriumPositionUnits=m  PySpringStiffness=0  PySpringStiffnessUnits=N/m  PyDampingCoefficient=world_damping  PyDampingCoefficientUnits=N/(m/s)  PyTorqueActuationMode=NoTorque  PyMotionActuationMode=ComputedMotion  PySensePosition=off  PySenseVelocity=off  PySenseAcceleration=off  PySenseTorqueForce=off  PySenseLowerLimitTorqueForce=off  PySenseUpperLimitTorqueForce=off  PyLowerLimitSpecify=off  PyLowerLimitBound=-1  PyLowerLimitBoundUnits=m  PyLowerLimitStiffness=1e6  PyLowerLimitStiffnessUnits=N/m  PyLowerLimitDamping=1e3  PyLowerLimitDampingUnits=N/(m/s)  PyLowerLimitTransitionRegionWidth=1e-4  PyLowerLimitTransitionRegionWidthUnits=m  PyUpperLimitSpecify=off  PyUpperLimitBound=1  PyUpperLimitBoundUnits=m  PyUpperLimitStiffness=1e6  PyUpperLimitStiffnessUnits=N/m  PyUpperLimitDamping=1e3  PyUpperLimitDampingUnits=N/(m/s)  PyUpperLimitTransitionRegionWidth=1e-4  PyUpperLimitTransitionRegionWidthUnits=m  PyPositionTargetSpecify=on  PyPositionTargetPriority=High  PyPositionTargetValue=0  PyPositionTargetValueUnits=m  PyVelocityTargetSpecify=off  PyVelocityTargetPriority=High  PyVelocityTargetValue=0  PyVelocityTargetValueUnits=m/s  PzEquilibriumPosition=0  PzEquilibriumPositionUnits=m  PzSpringStiffness=0  PzSpringStiffnessUnits=N/m  PzDampingCoefficient=world_damping  PzDampingCoefficientUnits=N/(m/s)  PzTorqueActuationMode=NoTorque  PzMotionActuationMode=ComputedMotion  PzSensePosition=off  PzSenseVelocity=off  PzSenseAcceleration=off  PzSenseTorqueForce=off  PzSenseLowerLimitTorqueForce=off  PzSenseUpperLimitTorqueForce=off  PzLowerLimitSpecify=off  PzLowerLimitBound=-1  PzLowerLimitBoundUnits=m  PzLowerLimitStiffness=1e6  PzLowerLimitStiffnessUnits=N/m  PzLowerLimitDamping=1e3  PzLowerLimitDampingUnits=N/(m/s)  PzLowerLimitTransitionRegionWidth=1e-4  PzLowerLimitTransitionRegionWidthUnits=m  PzUpperLimitSpecify=off  PzUpperLimitBound=1  PzUpperLimitBoundUnits=m  PzUpperLimitStiffness=1e6  PzUpperLimitStiffnessUnits=N/m  PzUpperLimitDamping=1e3  PzUpperLimitDampingUnits=N/(m/s)  PzUpperLimitTransitionRegionWidth=1e-4  PzUpperLimitTransitionRegionWidthUnits=m  PzPositionTargetSpecify=on  PzPositionTargetPriority=High  PzPositionTargetValue=init_height  PzPositionTargetValueUnits=cm  PzVelocityTargetSpecify=off  PzVelocityTargetPriority=High  PzVelocityTargetValue=0  PzVelocityTargetValueUnits=m/s  SphDefPosRotationMethod=None  SphDefPosRotationAngleUnits=deg  SphDefPosRotationStandardAxis=+Z  SphDefPosRotationAngle=0.0  SphDefPosRotationArbitraryAxis=[0 0 1]  SphDefPosFollAlignAxisA=+X  SphDefPosBaseAlignAxisA=+Y  SphDefPosFollAlignAxisB=+Y  SphDefPosBaseAlignAxisB=+Z  SphDefPosRotationSequenceAxes=FollowerAxes  SphDefPosRotationSequence=XYX  SphDefPosRotationSequenceAngles=[0 0 0]  SphDefPosRotationSequenceAnglesUnits=deg  SphDefPosRotationMatrix=[1 0 0; 0 1 0; 0 0 1]  SphEqPosRotationMethod=None  SphEqPosRotationAngleUnits=deg  SphEqPosRotationStandardAxis=+Z  SphEqPosRotationAngle=0.0  SphEqPosRotationArbitraryAxis=[0 0 1]  SphEqPosFollAlignAxisA=+X  SphEqPosBaseAlignAxisA=+Y  SphEqPosFollAlignAxisB=+Y  SphEqPosBaseAlignAxisB=+Z  SphEqPosRotationSequenceAxes=FollowerAxes  SphEqPosRotationSequence=XYX  SphEqPosRotationSequenceAngles=[0 0 0]  SphEqPosRotationSequenceAnglesUnits=deg  SphEqPosRotationMatrix=[1 0 0; 0 1 0; 0 0 1]  SphSpringStiffness=0  SphSpringStiffnessUnits=N*m/deg  SphDampingCoefficient=world_rot_damping  SphDampingCoefficientUnits=N*m/(rad/s)  SphActuateTorqueX=off  SphActuateTorqueY=off  SphActuateTorqueZ=off  SphActuateTorque=off  SphTorqueActuationMode=NoTorque  SphMotionActuationMode=ComputedMotion  SphActuationFrame=BaseFrame  SphSensePosition=off  SphSenseVelocityX=off  SphSenseVelocityY=off  SphSenseVelocityZ=off  SphSenseVelocity=off  SphSenseAccelerationX=off  SphSenseAccelerationY=off  SphSenseAccelerationZ=off  SphSenseAcceleration=off  SphSenseTorqueX=off  SphSenseTorqueY=off  SphSenseTorqueZ=off  SphSenseTorqueForce=off  SphSenseLowerLimitTorqueMag=off  SphSenseUpperLimitTorqueMag=off  SphSensingFrame=BaseFrame  SphLowerLimitSpecify=off  SphLowerLimitBound=15  SphLowerLimitBoundUnits=deg  SphLowerLimitStiffness=1e4  SphLowerLimitStiffnessUnits=N*m/deg  SphLowerLimitDamping=10  SphLowerLimitDampingUnits=N*m/(deg/s)  SphLowerLimitTransitionRegionWidth=0.1  SphLowerLimitTransitionRegionWidthUnits=deg  SphUpperLimitSpecify=off  SphUpperLimitBound=45  SphUpperLimitBoundUnits=deg  SphUpperLimitStiffness=1e4  SphUpperLimitStiffnessUnits=N*m/deg  SphUpperLimitDamping=10  SphUpperLimitDampingUnits=N*m/(deg/s)  SphUpperLimitTransitionRegionWidth=0.1  SphUpperLimitTransitionRegionWidthUnits=deg  SphPositionTargetRotationMethod=None  SphPositionTargetRotationAngleUnits=deg  SphPositionTargetRotationStandardAxis=+Z  SphPositionTargetRotationAngle=0.0  SphPositionTargetRotationArbitraryAxis=[0 0 1]  SphPositionTargetFollAlignAxisA=+X  SphPositionTargetBaseAlignAxisA=+Y  SphPositionTargetFollAlignAxisB=+Y  SphPositionTargetBaseAlignAxisB=+Z  SphPositionTargetRotationSequenceAxes=FollowerAxes  SphPositionTargetRotationSequence=XYX  SphPositionTargetRotationSequenceAngles=[0 0 0]  SphPositionTargetRotationSequenceAnglesUnits=deg  SphPositionTargetRotationMatrix=eye(3)  SphPositionTargetSpecify=off  SphPositionTargetPriority=High  SphVelocityTargetValue=[0 0 0]  SphVelocityTargetValueUnits=deg/s  SphVelocityTargetSpecify=off  SphVelocityTargetPriority=High  SphVelocityTargetInFollowerFrame=on
  Left Hip to Torso : sm_lib/Frames and Transforms/Rigid Transform  TranslationMethod=Cartesian  TranslationStandardOffset=0  TranslationLengthUnit=cm  TranslationStandardAxis=+Z  TranslationCartesianOffset=[torso_offset_x torso_y/2 torso_offset_z]  TranslationROffset=0  TranslationROffsetUnits=m  TranslationZOffset=0  TranslationZOffsetUnits=m  TranslationThetaOffset=0  TranslationThetaOffsetUnits=deg  RotationMethod=None  RotationAngleUnits=deg  RotationStandardAxis=+Z  RotationAngle=0.0  RotationArbitraryAxis=[0 0 1]  FollAlignAxisA=+X  BaseAlignAxisA=+Y  FollAlignAxisB=+Y  BaseAlignAxisB=+Z  RotationSequenceAxes=FollowerAxes  RotationSequence=XYX  RotationSequenceAngles=[0 0 0]  RotationSequenceAnglesUnits=deg  RotationMatrix=[1 0 0; 0 1 0; 0 0 1]
  Right Hip to Torso : sm_lib/Frames and Transforms/Rigid Transform  TranslationMethod=Cartesian  TranslationStandardOffset=0  TranslationLengthUnit=cm  TranslationStandardAxis=+Z  TranslationCartesianOffset=[torso_offset_x -torso_y/2 torso_offset_z]  TranslationROffset=0  TranslationROffsetUnits=m  TranslationZOffset=0  TranslationZOffsetUnits=m  TranslationThetaOffset=0  TranslationThetaOffsetUnits=deg  RotationMethod=None  RotationAngleUnits=deg  RotationStandardAxis=+Z  RotationAngle=0.0  RotationArbitraryAxis=[0 0 1]  FollAlignAxisA=+X  BaseAlignAxisA=+Y  FollAlignAxisB=+Y  BaseAlignAxisB=+Z  RotationSequenceAxes=FollowerAxes  RotationSequence=XYX  RotationSequenceAngles=[0 0 0]  RotationSequenceAnglesUnits=deg  RotationMatrix=[1 0 0; 0 1 0; 0 0 1]
  Robot Joint Controller : Subsystem  Variant=on
  Robot Leg L : Subsystem
  Robot Leg R : Subsystem
  Sensors : Subsystem
  Torso : sm_lib/Body Elements/Brick Solid  GraphicAmbientColor=[0.15 0.15 0.15 1.0]  BasedOnType=Density  BrickDimensions=[torso_x torso_y torso_z]  BrickDimensionUnits=cm  CenterOfMass=[0 0 0]  CenterOfMassUnits=m  GraphicDiffuseColor=[0.5 0.5 0.5]  Density=density  DensityUnits=kg/m^3  DoExposeReferenceFrame=on  GraphicEmissiveColor=[0.0 0.0 0.0 1.0]  ExportEntireGeometry=off  SerializedFrames=<Frames/>  MarkerShape=Sphere  MarkerSize=10  GraphicType=FromGeometry  InertiaType=CalculateFromGeometry  Mass=1  MassUnits=kg  MomentsOfInertia=[1 1 1]  MomentsOfInertiaUnits=kg*m^2  GraphicOpacity=1.0  ProductsOfInertia=[1 1 1]  ProductsOfInertiaUnits=kg*m^2  GraphicShininess=75  GraphicSpecularColor=[0.5 0.5 0.5 1.0]  GraphicVisPropType=SimpleVisualProperties
  Trajectory Display : sm_lib/Curves and Surfaces/Spline  GraphicAmbientColor=[0.15 0.15 0.15 1.0]  GraphicDiffuseColor=[0 0 0]  DataPoints=interPts  DataPointsUnits=m  GraphicEmissiveColor=[0.0 0.0 0.0 1.0]  EndConditionType=Natural  MarkerShape=Sphere  MarkerSize=10  GraphicType=FromGeometry  GraphicOpacity=1.0  GraphicShininess=75  GraphicSpecularColor=[0.5 0.5 0.5 1.0]  GraphicVisPropType=SimpleVisualProperties
      settings: SourceProductName=Simscape Multibody
  World and Ground : Subsystem
  measR : Outport  VectorParamsAs1DForOutWhenUnconnected=off
  measL : Outport  Port=2  VectorParamsAs1DForOutWhenUnconnected=off
  measBody : Outport  Port=3  VectorParamsAs1DForOutWhenUnconnected=off
  wires:
  Robot Leg L/1(meas) -> Robot Joint Controller/4(measL), measL/1
  Robot Leg R/1(meas) -> Robot Joint Controller/3(measR), measR/1
  angsR/1 -> Robot Joint Controller/1(refR)
  angsL/1 -> Robot Joint Controller/2(refL)
  Sensors/1(meas) -> measBody/1
  Robot Joint Controller/1(InputR) -> Robot Leg R/1(angs)
  Robot Joint Controller/2(InputL) -> Robot Leg L/1(angs)
  connections:
  Robot Leg R/RConn1 -- Right Hip to Torso/RConn1
  Robot Leg L/RConn1 -- Left Hip to Torso/RConn1
  Right Hip to Torso/LConn1 -- Sensors/RConn1 -- Left Hip to Torso/LConn1 -- Torso/RConn1 -- 6-DOF Joint/RConn1
  World and Ground/LConn1 -- Trajectory Display/LConn1 -- Sensors/LConn1 -- 6-DOF Joint/LConn1
  Robot Leg R/RConn2 -- World and Ground/RConn1 -- Robot Leg L/RConn2

== system walkingRobotUtils/Package Measurements 3D/Extract Measurements ==
  meas : Inport
  Bus Selector : BusSelector  OutputSignals=angle,speed,torque
  angle : Outport  VectorParamsAs1DForOutWhenUnconnected=off
  speed : Outport  Port=2  VectorParamsAs1DForOutWhenUnconnected=off
  torque : Outport  Port=3  VectorParamsAs1DForOutWhenUnconnected=off
  wires:
  Bus Selector/2 -> speed/1  "<speed>"
  Bus Selector/1 -> angle/1  "<angle>"
  meas/1 -> Bus Selector/1
  Bus Selector/3 -> torque/1  "<torque>"

== system walkingRobotUtils/Package Measurements 3D/Extract Measurements1 ==
  meas : Inport
  Bus Selector : BusSelector  OutputSignals=angle,speed,torque
  angle : Outport  VectorParamsAs1DForOutWhenUnconnected=off
  speed : Outport  Port=2  VectorParamsAs1DForOutWhenUnconnected=off
  torque : Outport  Port=3  VectorParamsAs1DForOutWhenUnconnected=off
  wires:
  Bus Selector/3 -> torque/1  "<torque>"
  meas/1 -> Bus Selector/1
  Bus Selector/1 -> angle/1  "<angle>"
  Bus Selector/2 -> speed/1  "<speed>"

== system walkingRobotUtils/Package Measurements 3D/Extract Measurements2 ==
  meas : Inport
  Bus Selector : BusSelector  OutputSignals=angle,speed,torque
  angle : Outport  VectorParamsAs1DForOutWhenUnconnected=off
  speed : Outport  Port=2  VectorParamsAs1DForOutWhenUnconnected=off
  torque : Outport  Port=3  VectorParamsAs1DForOutWhenUnconnected=off
  wires:
  Bus Selector/2 -> speed/1  "<speed>"
  Bus Selector/1 -> angle/1  "<angle>"
  meas/1 -> Bus Selector/1
  Bus Selector/3 -> torque/1  "<torque>"

== system walkingRobotUtils/Package Measurements 3D/Extract Measurements3 ==
  meas : Inport
  Bus Selector : BusSelector  OutputSignals=angle,speed,torque
  angle : Outport  VectorParamsAs1DForOutWhenUnconnected=off
  speed : Outport  Port=2  VectorParamsAs1DForOutWhenUnconnected=off
  torque : Outport  Port=3  VectorParamsAs1DForOutWhenUnconnected=off
  wires:
  Bus Selector/3 -> torque/1  "<torque>"
  meas/1 -> Bus Selector/1
  Bus Selector/1 -> angle/1  "<angle>"
  Bus Selector/2 -> speed/1  "<speed>"

== system walkingRobotUtils/Package Measurements 3D/Extract Measurements4 ==
  meas : Inport
  Bus Selector : BusSelector  OutputSignals=angle,speed,torque
  angle : Outport  VectorParamsAs1DForOutWhenUnconnected=off
  speed : Outport  Port=2  VectorParamsAs1DForOutWhenUnconnected=off
  torque : Outport  Port=3  VectorParamsAs1DForOutWhenUnconnected=off
  wires:
  Bus Selector/2 -> speed/1  "<speed>"
  Bus Selector/1 -> angle/1  "<angle>"
  meas/1 -> Bus Selector/1
  Bus Selector/3 -> torque/1  "<torque>"

== system walkingRobotUtils/Package Measurements 2D/Extract Measurements ==
  meas : Inport
  Bus Selector : BusSelector  OutputSignals=angle,speed,torque
  angle : Outport  VectorParamsAs1DForOutWhenUnconnected=off
  speed : Outport  Port=2  VectorParamsAs1DForOutWhenUnconnected=off
  torque : Outport  Port=3  VectorParamsAs1DForOutWhenUnconnected=off
  wires:
  Bus Selector/2 -> speed/1  "<speed>"
  Bus Selector/3 -> torque/1  "<torque>"
  meas/1 -> Bus Selector/1
  Bus Selector/1 -> angle/1  "<angle>"

== system walkingRobotUtils/Package Measurements 2D/Extract Measurements1 ==
  meas : Inport
  Bus Selector : BusSelector  OutputSignals=angle,speed,torque
  angle : Outport  VectorParamsAs1DForOutWhenUnconnected=off
  speed : Outport  Port=2  VectorParamsAs1DForOutWhenUnconnected=off
  torque : Outport  Port=3  VectorParamsAs1DForOutWhenUnconnected=off
  wires:
  Bus Selector/1 -> angle/1  "<angle>"
  meas/1 -> Bus Selector/1
  Bus Selector/3 -> torque/1  "<torque>"
  Bus Selector/2 -> speed/1  "<speed>"

== system walkingRobotUtils/Package Measurements 2D/Extract Measurements2 ==
  meas : Inport
  Bus Selector : BusSelector  OutputSignals=angle,speed,torque
  angle : Outport  VectorParamsAs1DForOutWhenUnconnected=off
  speed : Outport  Port=2  VectorParamsAs1DForOutWhenUnconnected=off
  torque : Outport  Port=3  VectorParamsAs1DForOutWhenUnconnected=off
  wires:
  Bus Selector/2 -> speed/1  "<speed>"
  Bus Selector/3 -> torque/1  "<torque>"
  meas/1 -> Bus Selector/1
  Bus Selector/1 -> angle/1  "<angle>"

== system walkingRobotUtils/Package Measurements/Extract Measurements ==
  meas : Inport
  Bus Selector : BusSelector  OutputSignals=angle,torque
  angle : Outport  VectorParamsAs1DForOutWhenUnconnected=off
  torque : Outport  Port=2  VectorParamsAs1DForOutWhenUnconnected=off
  wires:
  Bus Selector/2 -> torque/1  "<torque>"
  meas/1 -> Bus Selector/1
  Bus Selector/1 -> angle/1  "<angle>"

== system walkingRobotUtils/Robot Joint/Motion ==
  Joint : Inport
  Bus Creator : BusCreator  Inputs=3
  PS-Simulink Converter : nesl_utility/PS-Simulink Converter  PhysicalDomain=network_engine_domain  SubClassName=ps_output  LeftPortType=input  RightPortType=output  PseudoPeriodic=off  Frequencies=[]  Unit=1  AffineConversion=off
  PS-Simulink Converter1 : nesl_utility/PS-Simulink Converter  PhysicalDomain=network_engine_domain  SubClassName=ps_output  LeftPortType=input  RightPortType=output  PseudoPeriodic=off  Frequencies=[]  Unit=1  AffineConversion=off
  PS-Simulink Converter2 : nesl_utility/PS-Simulink Converter  PhysicalDomain=network_engine_domain  SubClassName=ps_output  LeftPortType=input  RightPortType=output  PseudoPeriodic=off  Frequencies=[]  Unit=1  AffineConversion=off
  Revolute Joint : sm_lib/Joints/Revolute Joint  JointMode=Normal  SenseConstraintForce=off  SenseConstraintForceX=off  SenseConstraintForceY=off  SenseConstraintForceZ=off  SenseConstraintTorque=off  SenseConstraintTorqueX=off  SenseConstraintTorqueY=off  SenseConstraintTorqueZ=off  SenseTotalForce=off  SenseTotalForceX=off  SenseTotalForceY=off  SenseTotalForceZ=off  SenseTotalTorque=off  SenseTotalTorqueX=off  SenseTotalTorqueY=off  SenseTotalTorqueZ=off  CompositeWrenchDir=FollowerOnBase  CompositeWrenchFrame=BaseFrame  EquilibriumPosition=0  EquilibriumPositionUnits=deg  SpringStiffness=0  SpringStiffnessUnits=N*m/deg  DampingCoefficient=jointDamping  DampingCoefficientUnits=N*m/(rad/s)  TorqueActuationMode=ComputedTorque  MotionActuationMode=InputMotion  SensePosition=on  SenseVelocity=on  SenseAcceleration=off  SenseTorqueForce=on  SenseLowerLimitTorqueForce=off  SenseUpperLimitTorqueForce=off  LowerLimitSpecify=on  LowerLimitBound=lowerLimit  LowerLimitBoundUnits=rad  LowerLimitStiffness=limitK  LowerLimitStiffnessUnits=N*m/rad  LowerLimitDamping=limitD  LowerLimitDampingUnits=N*m/(rad/s)  LowerLimitTransitionRegionWidth=0.1  LowerLimitTransitionRegionWidthUnits=deg  UpperLimitSpecify=on  UpperLimitBound=upperLimit  UpperLimitBoundUnits=rad  UpperLimitStiffness=limitK  UpperLimitStiffnessUnits=N*m/rad  UpperLimitDamping=limitD  UpperLimitDampingUnits=N*m/(rad/s)  UpperLimitTransitionRegionWidth=0.1  UpperLimitTransitionRegionWidthUnits=deg  PositionTargetSpecify=on  PositionTargetPriority=High  PositionTargetValue=initAngle  PositionTargetValueUnits=rad  VelocityTargetSpecify=off  VelocityTargetPriority=High  VelocityTargetValue=0  VelocityTargetValueUnits=deg/s
  Simulink-PS Converter : nesl_utility/Simulink-PS Converter  PhysicalDomain=network_engine_domain  SubClassName=ps_input  LeftPortType=input  RightPortType=output  PseudoPeriodic=off  Frequencies=[]  NoiseDistribution=none  NoiseParameters=[]  Unit=1  AffineConversion=off  FilteringAndDerivatives=filter  SimscapeFilterOrder=2  InputFilterTimeConstant=motion_time_constant  UdotUserProvided=0
  F : PMIOPort  Side=Right
  B : PMIOPort  Port=2  Side=Left
  Sensor : Outport  VectorParamsAs1DForOutWhenUnconnected=off
  wires:
  PS-Simulink Converter2/1 -> Bus Creator/1  "torque"
  Bus Creator/1 -> Sensor/1
  PS-Simulink Converter1/1 -> Bus Creator/2  "angle"
  PS-Simulink Converter/1 -> Bus Creator/3  "speed"
  Joint/1 -> Simulink-PS Converter/1  "motion"
  connections:
  Revolute Joint/RConn4 -- PS-Simulink Converter2/LConn1
  Revolute Joint/RConn1 -- F/RConn1
  PS-Simulink Converter/LConn1 -- Revolute Joint/RConn3
  Simulink-PS Converter/RConn1 -- Revolute Joint/LConn2
  Revolute Joint/RConn2 -- PS-Simulink Converter1/LConn1
  Revolute Joint/LConn1 -- B/RConn1
